simulink model "pilot_command"  (R2016b)
settings: Solver=FixedStepAuto  StartTime=0.0  StopTime=inf  FixedStep=0.05  RelTol=1e-3
undefined symbols (not defined in the file): sigbuilder_block
libraries: simulink x4, xpcutilitieslib x1, slrtlib x1, aerolibanimutils x1, instrumentlib x1
settings Model: Creator=Florian Wachter  LastModifiedBy=Florian Wachter

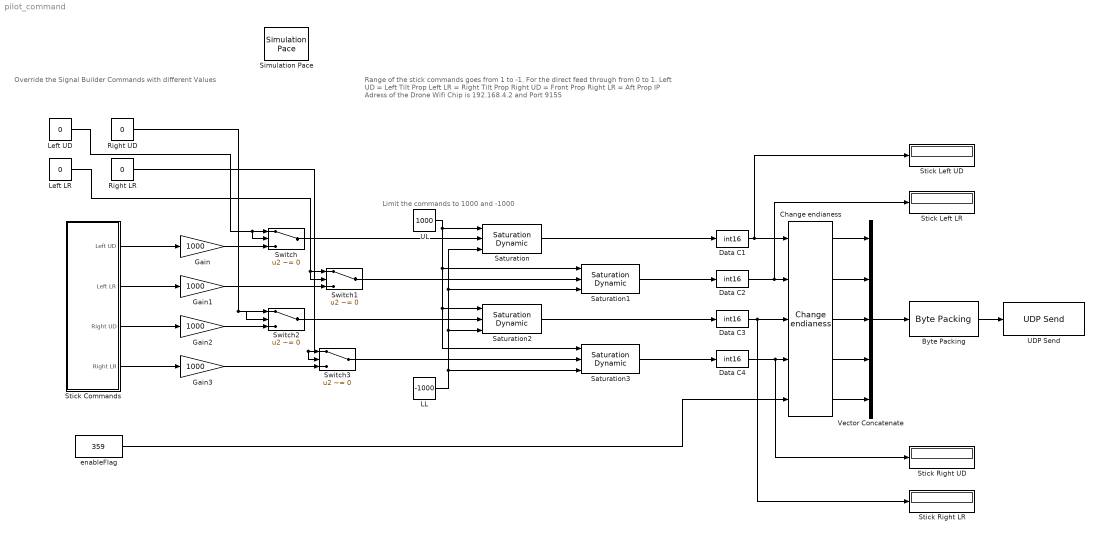
== system pilot_command ==
  note: Limit the commands to 1000 and -1000
  note: Range of the stick commands goes from 1 to -1. For the direct feed
      | through from 0 to 1.
      | Left UD = Left Tilt Prop
      | Left LR = Right Tilt Prop
      | Right UD = Front Prop
      | Right LR = Aft Prop
      | IP Adress of the Drone Wifi Chip is 192.168.4.2 and Port 9155
  note: Override the Signal Builder Commands with
      | different Values
  "Byte Packing " : xpcutilitieslib/Byte Packing   MaskPackedDataType=int16  MaskUnpackedDataTypes={'int16'}  MaskAlignment=1
  "Change endianess " : slrtlib/Shared Memory/Change endianess   numInp=5  lengthIn=Byte
  Data C{1..4} (4 alike) : DataTypeConversion  OutDataTypeStr=int16  RndMeth=Nearest
  Gain{,1..3} (4 alike) : Gain  Gain=1000
  LL : Constant  Value=-1000
  Left LR : Constant  Value=0  OutMin=-1000  OutMax=1000  OutDataTypeStr=int16
  Left UD : Constant  Value=0  OutMin=-1000  OutMax=1000  OutDataTypeStr=int16
  Right LR : Constant  Value=0  OutMin=-1000  OutMax=1000  OutDataTypeStr=int16
  Right UD : Constant  Value=0  OutMin=-1000  OutMax=1000  OutDataTypeStr=int16
  Saturation{,1..3} (4 alike) : simulink/Discontinuities/Saturation Dynamic  OutMin=[]  OutMax=[]  OutDataTypeStr=Inherit: Same as second input  OutDataType=fixdt(1, 16)  OutScaling=2^-10  DoSatur=off
  Simulation Pace : aerolibanimutils/Simulation Pace  SimulationPace=1/4  SleepMode=MATLAB Thread  OutputPaceError=off  SampleTime=1/20
  Stick Commands : Subsystem  Tag=STV Subsys  LoadFcn=sigbuilder_block('load');  StartFcn=sigbuilder_block('start');  StopFcn=sigbuilder_block('stop');  ClipboardFcn=sigbuilder_block('clipboard');  mask(Sigbuilder block){tuvar=[0:10]}
      mask help: Simulink:masks:SigbuilderBlock_MD
      mask init:
      | if ~strcmp(get_param(bdroot(gcbh),'SimulationStatus'),'stopped') tuvar = sigbuilder_block('maskInit'); end
      settings: CopyFcn=sigbuilder_block('copy');  DeleteFcn=sigbuilder_block('delete');  ModelCloseFcn=sigbuilder_block('modelClose');  PreSaveFcn=sigbuilder_block('preSave');  PauseFcn=sigbuilder_block('pause');  ContinueFcn=sigbuilder_block('continue');  NameChangeFcn=sigbuilder_block('namechange');  OpenFcn=sigbuilder_block('open',[6 33 948 637.5 ]);  CloseFcn=sigbuilder_block('close');
      mask Display: plot(0, 0, 100, 100,[2, 2, 32, 32, 2], [68, 8, 8, 68, 68],[32, 2], [38, 38], [32, 19, 2],[53, 60, 44], [32, 17, 17, 2],[16, 16, 31, 31]);txt = getActiveGroup(gcbh);text(2, 100, txt,'verticalAlignment', 'top');
  Stick Left LR : Display
  Stick Left UD : Display
  Stick Right LR : Display
  Stick Right UD : Display
  Switch{,1..3} (4 alike) : Switch  Criteria=u2 ~= 0
  UDP Send : instrumentlib/UDP Send  Host=192.168.4.3  Port=9155  LocalPort=-1  EnableBlockingMode=off  ByteOrder=BigEndian
  UL : Constant  Value=1000
  Vector Concatenate : Concatenate  NumInputs=5
  enableFlag : Constant  Value=359  OutDataTypeStr=int16
  wires:
  Vector Concatenate/1 -> "Byte Packing "/1
  "Byte Packing "/1 -> UDP Send/1
  Switch/1 -> Saturation/2
  Switch1/1 -> Saturation1/2
  Switch2/1 -> Saturation2/2
  Switch3/1 -> Saturation3/2
  Gain/1 -> Switch/3
  Gain1/1 -> Switch1/3
  Gain2/1 -> Switch2/3
  Gain3/1 -> Switch3/3
  Data C1/1 -> Stick Left UD/1, "Change endianess "/1
  "Change endianess "/1 -> Vector Concatenate/1
  Data C2/1 -> Stick Left LR/1, "Change endianess "/2
  "Change endianess "/2 -> Vector Concatenate/2
  Data C3/1 -> Stick Right LR/1, "Change endianess "/3
  Data C4/1 -> Stick Right UD/1, "Change endianess "/4
  "Change endianess "/3 -> Vector Concatenate/3
  "Change endianess "/4 -> Vector Concatenate/4
  "Change endianess "/5 -> Vector Concatenate/5
  enableFlag/1 -> "Change endianess "/5
  Saturation1/1 -> Data C2/1
  Saturation2/1 -> Data C3/1
  Saturation3/1 -> Data C4/1
  Left UD/1 -> Switch/2, Switch/1
  Left LR/1 -> Switch1/2, Switch1/1
  Right UD/1 -> Switch2/2, Switch2/1
  Right LR/1 -> Switch3/2, Switch3/1
  Stick Commands/1(Left UD) -> Gain/1
  Stick Commands/2(Left LR) -> Gain1/1
  Stick Commands/3(Right UD) -> Gain2/1
  Stick Commands/4(Right LR) -> Gain3/1
  Saturation/1 -> Data C1/1
  LL/1 -> Saturation1/3, Saturation/3, Saturation2/3, Saturation3/3
  UL/1 -> Saturation/1, Saturation1/1, Saturation2/1, Saturation3/1

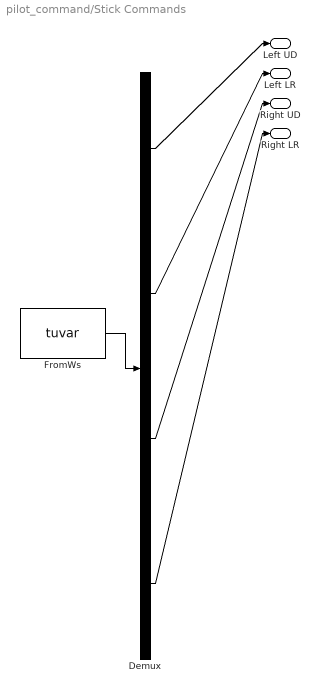
== system pilot_command/Stick Commands ==
  Demux : Demux  Tag=STV Demux
  FromWs : FromWorkspace  Tag=STV FromWs  VariableName=tuvar  SampleTime=0
      SigBuilderData=|
      | common.afterFinalStr = 'Extrapolate'
      | common.sampleTime = 0
      | dataSet(1).timeRange = [0 11]
      | dataSet(1).name = 'Group 1'
      | dataSet(2).timeRange = [0 10]
      | dataSet(2).name = 'Group 2'
      | dataSet(3).timeRange = [0 20]
      | dataSet(3).name = 'Group 3'
      | dataSet(4).timeRange = [0 10]
      | dataSet(4).name = 'Group 4'
      | dataSet(5).timeRange = [0 20]
      | dataSet(5).name = 'Group 5'
      | dataSet(6).timeRange = [0 11]
      | dataSet(6).name = 'Group 6'
      | dataSet(7).timeRange = [0 20]
      | dataSet(7).name = 'Group 7'
      | sbobj.Groups(1).Name = 'Group 1'
      | sbobj.Groups(1).Signals(1).Name = 'Left UD'
      | sbobj.Groups(1).Signals(1).XData = [0 11]
      | sbobj.Groups(1).Signals(1).YData = [0 0]
      | sbobj.Groups(1).Signals(2).Name = 'Left LR'
      | sbobj.Groups(1).Signals(2).XData = [0 11]
      | sbobj.Groups(1).Signals(2).YData = [0 0]
      | sbobj.Groups(1).Signals(3).Name = 'Right UD'
      | sbobj.Groups(1).Signals(3).XData = [0 1 1 2 2 3 3 4 4 5 5 6 6 7 7 8 8 9 9 10 11]
      | sbobj.Groups(1).Signals(3).YData = [0.1 0.1 0.2 0.2 0.3 0.3 0.4 0.4 0.5 0.5 0.6 0.6 0.7 0.7 0.8 0.8 0.9 0.9 1 1 0]
      | sbobj.Groups(1).Signals(4).Name = 'Right LR'
      | sbobj.Groups(1).Signals(4).XData = [0 1 1 2 2 3 3 4 4 5 5 6 6 7 7 8 8 9 9 10 11]
      | sbobj.Groups(1).Signals(4).YData = [0.1 0.1 0.2 0.2 0.3 0.3 0.4 0.4 0.5 0.5 0.6 0.6 0.7 0.7 0.8 0.8 0.9 0.9 1 1 0]
      | sbobj.Groups(1).TimeRange = [0 11]
      | sbobj.Groups(2).Name = 'Group 2'
      | sbobj.Groups(2).Signals(1).Name = 'Left UD'
      | sbobj.Groups(2).Signals(1).XData = [0 1 2 2.5 3 10]
      | sbobj.Groups(2).Signals(1).YData = [0 0 1 -1 0 0]
      | sbobj.Groups(2).Signals(2).Name = 'Left LR'
      | sbobj.Groups(2).Signals(2).XData = [0 3 4 4.5 5 10]
      | sbobj.Groups(2).Signals(2).YData = [0 0 1 -1 0 0]
      | sbobj.Groups(2).Signals(3).Name = 'Right UD'
      | sbobj.Groups(2).Signals(3).XData = [0 5 6 6.5 7 10]
      | sbobj.Groups(2).Signals(3).YData = [0 0 1 -1 0 0]
      | sbobj.Groups(2).Signals(4).Name = 'Right LR'
      | sbobj.Groups(2).Signals(4).XData = [0 7 8 8.5 9 10]
      | sbobj.Groups(2).Signals(4).YData = [0 0 1 -1 0 0]
      | sbobj.Groups(3).Name = 'Group 3'
      | sbobj.Groups(3).Signals(1).Name = 'Left UD'
      | sbobj.Groups(3).Signals(1).XData = [0 1 1 3 3 5 5 7 7 9 9 11 11 13 13 15 15 17 17 19 19 20]
      | sbobj.Groups(3).Signals(1).YData = [0 0 0.1 0.1 0.2 0.2 0.3 0.3 0.4 0.4 0.5 0.5 0.6 0.6 0.7 0.7 0.8 0.8 0.9 0.9 1 1]
      | sbobj.Groups(3).Signals(2).Name = 'Left LR'
      | sbobj.Groups(3).Signals(2).XData = [0 20]
      | sbobj.Groups(3).Signals(2).YData = [0 0]
      | sbobj.Groups(3).Signals(3).Name = 'Right UD'
      | sbobj.Groups(3).Signals(3).XData = [0 20]
      | sbobj.Groups(3).Signals(3).YData = [0 0]
      | sbobj.Groups(3).Signals(4).Name = 'Right LR'
      | sbobj.Groups(3).Signals(4).XData = [0 20]
      | sbobj.Groups(3).Signals(4).YData = [0 0]
      | sbobj.Groups(3).TimeRange = [0 20]
      | sbobj.Groups(4).Name = 'Group 4'
      | sbobj.Groups(4).Signals(1).Name = 'Left UD'
      | sbobj.Groups(4).Signals(1).XData = [0 10]
      | sbobj.Groups(4).Signals(1).YData = [0 1]
      | sbobj.Groups(4).Signals(2).Name = 'Left LR'
      | sbobj.Groups(4).Signals(2).XData = [0 10]
      | sbobj.Groups(4).Signals(2).YData = [0 1]
      | sbobj.Groups(4).Signals(3).Name = 'Right UD'
      | sbobj.Groups(4).Signals(3).XData = [0 10]
      | sbobj.Groups(4).Signals(3).YData = [0 1]
      | sbobj.Groups(4).Signals(4).Name = 'Right LR'
      | sbobj.Groups(4).Signals(4).XData = [0 10]
      | sbobj.Groups(4).Signals(4).YData = [0 0.981]
      | sbobj.Groups(5).Name = 'Group 5'
      | sbobj.Groups(5).Signals(1).Name = 'Left UD'
      | sbobj.Groups(5).Signals(1).XData = [0 1 2 2 3 3 4 4 5 5 6 7 7 8 8 9 9 10 10 11 11 12 12 13.1 13.1 14 14 20]
      | sbobj.Groups(5).Signals(1).YData = [0.1 0.1 0.1 0.2 0.2 0.3 0.3 0.4 0.4 0.5 0.525 0.525 0.55 0.55 0.575 0.575 0.6 0.6 0.625 0.625 0.65 0.65 0.675 0.675 0.7 0.7 0.7 0.01]
      | sbobj.Groups(5).Signals(2).Name = 'Left LR'
      | sbobj.Groups(5).Signals(2).XData = [0 1 2 2 3 3 4 4 5 5 6 7 7 8 8 9 9 10 10 11 11 12 12 13.1 13.1 14 14 20]
      | sbobj.Groups(5).Signals(2).YData = [0.1 0.1 0.1 0.2 0.2 0.3 0.3 0.4 0.4 0.5 0.525 0.525 0.55 0.55 0.575 0.575 0.6 0.6 0.625 0.625 0.65 0.65 0.675 0.675 0.7 0.7 0.7 0.01]
      | sbobj.Groups(5).Signals(3).Name = 'Right UD'
      | sbobj.Groups(5).Signals(3).XData = [0 1 2 2 3 3 4 4 5 5 6 7 7 8 8 9 9 10 10 11 11 12 12 13.1 13.1 14 14 20]
      | sbobj.Groups(5).Signals(3).YData = [0.1 0.1 0.1 0.2 0.2 0.3 0.3 0.4 0.4 0.5 0.525 0.525 0.55 0.55 0.575 0.575 0.6 0.6 0.625 0.625 0.65 0.65 0.675 0.675 0.7 0.7 0.7 0.01]
      | sbobj.Groups(5).Signals(4).Name = 'Right LR'
      | sbobj.Groups(5).Signals(4).XData = [0 1 2 2 3 3 4 4 5 5 6 7 7 8 8 9 9 10 10 11 11 12 12 13.1 13.1 14 14 20]
      | sbobj.Groups(5).Signals(4).YData = [0.1 0.1 0.1 0.2 0.2 0.3 0.3 0.4 0.4 0.5 0.525 0.525 0.55 0.55 0.575 0.575 0.6 0.6 0.625 0.625 0.65 0.65 0.675 0.675 0.7 0.7 0.7 0.01]
      | sbobj.Groups(5).TimeRange = [0 20]
      | sbobj.Groups(6).Name = 'Group 6'
      | sbobj.Groups(6).Signals(1).Name = 'Left UD'
      | sbobj.Groups(6).Signals(1).XData = [0 1 1 2 2 3 3 4 4 5 5 6 6 7 7 8 8 9 9 10 11]
      | sbobj.Groups(6).Signals(1).YData = [0.1 0.1 0.2 0.2 0.3 0.3 0.4 0.4 0.5 0.5 0.6 0.6 0.7 0.7 0.8 0.8 0.9 0.9 1 1 0]
      | sbobj.Groups(6).Signals(2).Name = 'Left LR'
      | sbobj.Groups(6).Signals(2).XData = [0 1 1 2 2 3 3 4 4 5 5 6 6 7 7 8 8 9 9 10 11]
      | sbobj.Groups(6).Signals(2).YData = [0.1 0.1 0.2 0.2 0.3 0.3 0.4 0.4 0.5 0.5 0.6 0.6 0.7 0.7 0.8 0.8 0.9 0.9 1 1 0]
      | sbobj.Groups(6).Signals(3).Name = 'Right UD'
      | sbobj.Groups(6).Signals(3).XData = [0 11]
      | sbobj.Groups(6).Signals(3).YData = [0 0]
      | sbobj.Groups(6).Signals(4).Name = 'Right LR'
      | sbobj.Groups(6).Signals(4).XData = [0 11]
      | sbobj.Groups(6).Signals(4).YData = [0 0]
      | sbobj.Groups(6).TimeRange = [0 11]
      | sbobj.Groups(7).Name = 'Group 7'
      | sbobj.Groups(7).Signals(1).Name = 'Left UD'
      | sbobj.Groups(7).Signals(1).XData = [0 1 2 2 3 3 4 4 5 5 6 6 7 7 8 8 9 9 10 11 20]
      | sbobj.Groups(7).Signals(1).YData = [0.1 0.1 0.1 0.2 0.2 0.4 0.4 0.5 0.5 0.6 0.6 0.7 0.7 0.8 0.8 0.9 0.9 1 1 0 0]
      | sbobj.Groups(7).Signals(2).Name = 'Left LR'
      | sbobj.Groups(7).Signals(2).XData = [0 1 1 2 2 3 3 4 4 5 5 6 6 7 7 8 8 9 9 10 11 20]
      | sbobj.Groups(7).Signals(2).YData = [0.1 0.1 0.2 0.2 0.3 0.3 0.4 0.4 0.5 0.5 0.6 0.6 0.7 0.7 0.8 0.8 0.9 0.9 1 1 0 0]
      | sbobj.Groups(7).Signals(3).Name = 'Right UD'
      | sbobj.Groups(7).Signals(3).XData = [0 1 1 2 2 3 3 4 4 5 5 6 6 7 7 8 8 9 9 10 11 20]
      | sbobj.Groups(7).Signals(3).YData = [0.1 0.1 0.2 0.2 0.3 0.3 0.4 0.4 0.5 0.5 0.6 0.6 0.7 0.7 0.8 0.8 0.9 0.9 1 1 0 0]
      | sbobj.Groups(7).Signals(4).Name = 'Right LR'
      | sbobj.Groups(7).Signals(4).XData = [0 1 1 2 2 3 3 4 4 5 5 6 6 7 7 8 8 9 9 10 11 20]
      | sbobj.Groups(7).Signals(4).YData = [0.1 0.1 0.2 0.2 0.3 0.3 0.4 0.4 0.5 0.5 0.6 0.6 0.7 0.7 0.8 0.8 0.9 0.9 1 1 0 0]
      | sbobj.Groups(7).TimeRange = [0 20]
  Left UD : Outport  Tag=STV Outport
  Left LR : Outport  Tag=STV Outport  Port=2
  Right UD : Outport  Tag=STV Outport  Port=3
  Right LR : Outport  Tag=STV Outport  Port=4
  wires:
  FromWs/1 -> Demux/1
  Demux/1 -> Left UD/1
  Demux/2 -> Left LR/1
  Demux/3 -> Right UD/1
  Demux/4 -> Right LR/1
